simulink model "PickAndPlace_Simulation_Simscape"  (R2024b)
settings: Solver=ode2  StartTime=0.0  StopTime=600  FixedStep=0.005  RelTol=1e-3
InitFcn:
  | qarmRigidBodyTree = importrobot('E:\Applied Robotics\project-ar\QARMS-Matlabs-main\resources\qarm\urdf\QARM.urdf');
  | qarmRigidBodyTree.Bodies{1,3}.Joint.PositionLimits(1) = -pi/4;
  | show(qarmRigidBodyTree);
undefined symbols (not defined in the file or in its folder): EFFECTOR, END, Levenberg, Marquardt, X, Y, Z
libraries: sm_lib x50, nesl_utility x9, robotmaniplib x2, quarc_library x1
(part 2 of 2)

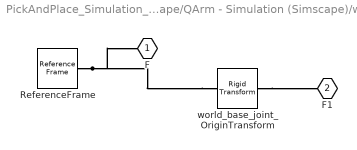
== system PickAndPlace_Simulation_Simscape/QArm - Simulation (Simscape)/world ==
  ReferenceFrame : sm_lib/Frames and Transforms/Reference Frame
  world_base_joint_OriginTransform : sm_lib/Frames and Transforms/Rigid Transform  RotationMethod=RotationSequence  FollAlignAxisA=+X  BaseAlignAxisA=+Y  FollAlignAxisB=+Y  BaseAlignAxisB=+Z  RotationStandardAxis=+Z  RotationAngle=0.0  RotationAngleUnits=deg  RotationArbitraryAxis=[0 0 1]  RotationSequenceAxes=BaseAxes  RotationSequence=XYZ  RotationSequenceAngles=[0, 0, 0]  RotationSequenceAnglesUnits=rad  RotationMatrix=[1 0 0; 0 1 0; 0 0 1]  Quaternion=[1 0 0 0]  TranslationMethod=Cartesian  TranslationCartesianOffset=[0, 0, 0]  TranslationCartesianOffsetUnits=m  TranslationStandardAxis=+Z  TranslationStandardOffset=0  TranslationStandardOffsetUnits=m  TranslationROffset=0  TranslationROffsetUnits=m  TranslationThetaOffset=0  TranslationThetaOffsetUnits=deg  TranslationZOffset=0  TranslationZOffsetUnits=m
  F : PMIOPort  Side=Left
  F1 : PMIOPort  Port=2  Side=Right
  connections:
  world_base_joint_OriginTransform/LConn1 -- ReferenceFrame/RConn1 -- F/RConn1
  world_base_joint_OriginTransform/RConn1 -- F1/RConn1

== matlab function PickAndPlace_Simulation_Simscape/MATLAB Function3 ==
  data: pos output; grip output
function [pos, grip] = gesture_control()

[pos, grip] = gesture_control_wrapper();

end

== matlab function PickAndPlace_Simulation_Simscape/MATLAB Function1 ==
  data: pos output; grip output
function [pos, grip] = manual_control

[pos, grip] = manual_wrapper();

end

== matlab function PickAndPlace_Simulation_Simscape/MATLAB Function ==
  data: fruitType output
function fruitType = fcn()

coder.extrinsic('py.yolo_simulink.detect_fruit');

fruitType = 0;  % double

result = py.yolo_simulink.detect_fruit();

fruitType = double(result);

end

== stateflow chart PickAndPlace_Simulation_Simscape/Chart ==
  state flag = closeEnough(a,b,t) [function]
  state Wait
    gripper=0;
    targetPosition=home;
  state Detect1
    detectedType = data;
  state GotoPick
    targetPosition=pick;
    flag = closeEnough(measPosition, targetPosition, threshold);
  state CloseGripper
    gripper=1;
  state GotoHome
    targetPosition=home;
    flag = closeEnough(measPosition, targetPosition, threshold);
  state OpenGripper
    gripper=0;
  state GotoPlace
    switch detectedType
    case 1
    targetPosition = place1;  % strawberry
    case 2
    targetPosition = place2;  % banana
    case 3
    targetPosition = place3;  % tomato
    end
    flag = closeEnough(measPosition, targetPosition, threshold);
  (default) -> Wait
  GotoPick -> Detect1 : [after(2,sec) && flag]
  Wait -> GotoPick : [start && after(2,sec)]
  Detect1 -> CloseGripper : [after(5,sec) && detectedType > 0]
  GotoHome -> GotoPick [order 2] : [after(2,sec) && flag]
  CloseGripper -> GotoHome : [after(2,sec)]
  GotoHome -> GotoPlace [order 1] : [gripper && after(2,sec) && flag]
  OpenGripper -> GotoHome : [after(2,sec)]
  GotoPlace -> OpenGripper : [after(3,sec) && flag]
  data: a function_input double size=[3,1]; b function_input double size=[3,1]; flag function_output; t function_input double size=[1]; start input; data input; place3 input; place2 input; pick input size=[3,1]; targetPosition output size=[3,1]; gripper output size=[1]; place1 input double size=[3,1]; home input double size=[3,1]; threshold input; measPosition input double size=[3,1]; flag local; detectedType local double
